simulink model "solarPressure_test"  (R2018b)
settings: Solver=VariableStepAuto  StartTime=0.0  StopTime=0  RelTol=1e-3
values from neighbouring files (symbols this model uses):
  utc_test = 137803367    [solarPressure_test_init.m]    (also in sunVector_test_init.m = 197208000)
undefined symbols (not defined in the file or in its folder): state
libraries: solarPressure_lib x1, time_lib x1
settings Model: Creator=devantormey  LastModifiedBy=devantormey

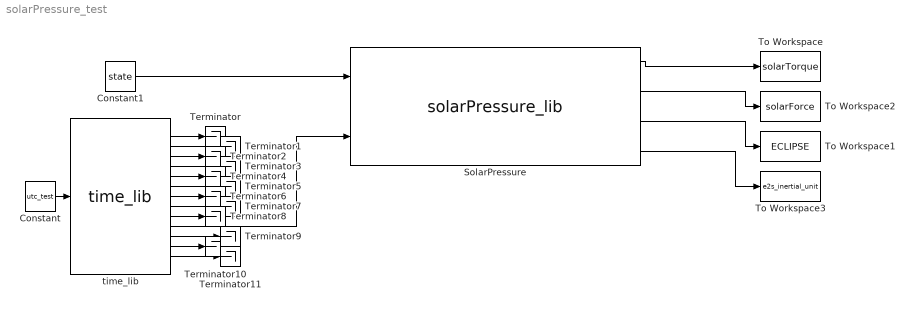
== system solarPressure_test ==
  Constant : Constant  Value=utc_test
  Constant1 : Constant  Value=state
  SolarPressure : solarPressure_lib/solarPressure_lib  SystemSampleTime=-1
  Terminator{,1..11} (12 alike) : Terminator
  To Workspace : ToWorkspace  VariableName=solarTorque  SaveFormat=Timeseries  SampleTime=-1
  To Workspace1 : ToWorkspace  VariableName=ECLIPSE  SaveFormat=Timeseries  SampleTime=-1
  To Workspace2 : ToWorkspace  VariableName=solarForce  SaveFormat=Timeseries  SampleTime=-1
  To Workspace3 : ToWorkspace  VariableName=e2s_inertial_unit  SaveFormat=Timeseries  SampleTime=-1
  "time_lib " : time_lib/time_lib    SystemSampleTime=-1
  wires:
  Constant/1 -> "time_lib "/1
  SolarPressure/1 -> To Workspace/1
  "time_lib "/10 -> SolarPressure/2
  "time_lib "/1 -> Terminator/1
  "time_lib "/2 -> Terminator1/1
  "time_lib "/3 -> Terminator2/1
  "time_lib "/4 -> Terminator3/1
  "time_lib "/5 -> Terminator4/1
  "time_lib "/6 -> Terminator5/1
  "time_lib "/7 -> Terminator6/1
  "time_lib "/8 -> Terminator7/1
  "time_lib "/9 -> Terminator8/1
  "time_lib "/11 -> Terminator9/1
  "time_lib "/12 -> Terminator10/1
  "time_lib "/13 -> Terminator11/1
  SolarPressure/2 -> To Workspace2/1
  Constant1/1 -> SolarPressure/1
  SolarPressure/3 -> To Workspace1/1
  SolarPressure/4 -> To Workspace3/1
